simulink model "controle_pid"  (R2018b)
settings: Solver=VariableStepAuto  StartTime=0.0  StopTime=800  RelTol=1e-3
values from neighbouring files (symbols this model uses):
  h10 = 25    [dadosTanque.m]
  h20 = 20    [dadosTanque.m]
  k1 = 25    [dadosTanque.m]
  k2 = 25    [dadosTanque.m]
  kac = 20    [dadosTanque.m]
  Ki = blkdiag(Ki,1/tau(i))    [calcula_parametros_PID.m]
  Kp = blkdiag(Kp, 0.6*tau(i)/(k(i)*theta(i)))    [calcula_parametros_PID.m]
  q10 = k1*sqrt(h10) + kac*sqrt(h10-h20)    [dadosTanque.m]
  q20 = k2*sqrt(h20) - kac*sqrt(h10-h20)    [dadosTanque.m]
  sw_anti_windup = 1    [simula_anti_windup.m]    (also in simula_d_filter.m; simula_noise.m; simula_pid.m = 0)
  sw_d_filter = 0    [simula_anti_windup.m]    (also in simula_d_filter.m = 1; simula_noise.m; simula_pid.m)
  sw_noise = 0    [simula_anti_windup.m]    (also in simula_d_filter.m = 1; simula_div_acao_pond.m = 1; simula_div_acao_pond2.m = 1; simula_div_acao_trad.m = 1)
  Td = blkdiag(Td,theta(i)/2)    [calcula_parametros_PID.m]
settings Model: Creator=Caléo  LastModifiedBy=Caléo
settings SolverCC: ZeroCrossAlgorithm=Adaptive
settings DebuggingCC: IgnoredZcDiagnostic=none

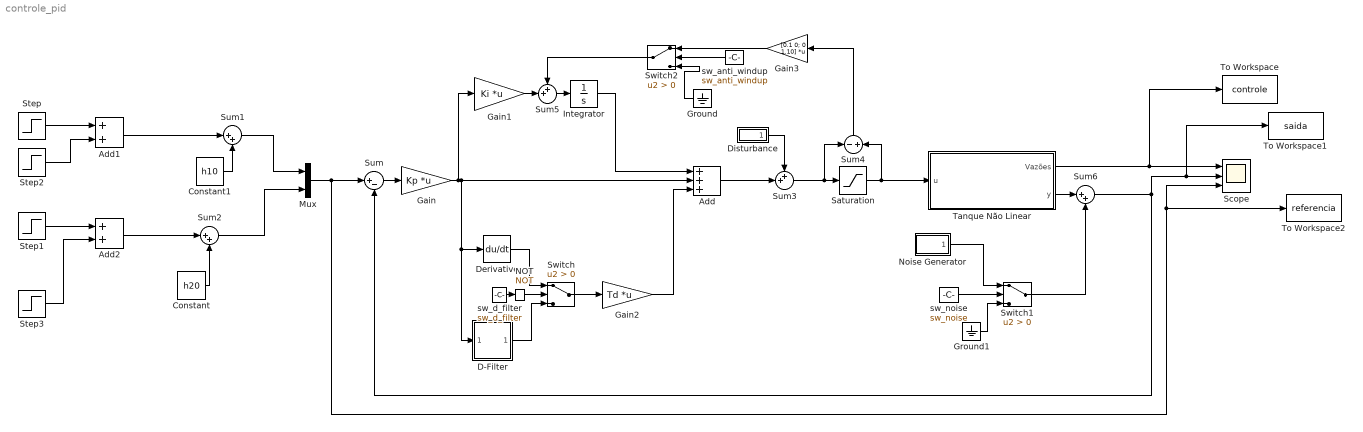
== system controle_pid ==
  Add : Sum  Inputs=+++
  Add1 : Sum
  Add2 : Sum
  Constant : Constant  Value=h20
  Constant1 : Constant  Value=h10
  D-Filter : Subsystem
  Derivative : Derivative
  Disturbance : Subsystem
  Gain : Gain  Gain=Kp  Multiplication=Matrix(K*u)
  Gain1 : Gain  Gain=Ki  Multiplication=Matrix(K*u)
  Gain2 : Gain  Gain=Td  Multiplication=Matrix(K*u)
  Gain3 : Gain  Gain=[0.1 0; 0 1.10]  Multiplication=Matrix(K*u)
  Ground : Ground
  Ground1 : Ground
  Integrator : Integrator
  Mux : Mux  Inputs=2
  NOT : Logic  Operator=NOT  IconShape=distinctive  AllPortsSameDT=off  OutDataTypeStr=boolean
  Noise Generator : Subsystem
  Saturation : Saturate  UpperLimit=[0.2*q10 0.2*q20]  LowerLimit=[-q10 ;-q20]
  Scope : Scope  NumInputPorts=3
  Step : Step  After=5  SampleTime=0
  Step1 : Step  After=3  SampleTime=0
  Step2 : Step  Time=300  After=-6  SampleTime=0
  Step3 : Step  Time=300  After=-6  SampleTime=0
  Sum : Sum  Inputs=|+-
  Sum1 : Sum  Inputs=|++
  Sum2 : Sum  Inputs=|++
  Sum3 : Sum  Inputs=++|
  Sum4 : Sum  Inputs=-+
  Sum5 : Sum  Inputs=++|
  Sum6 : Sum  Inputs=|++
  Switch : Switch  Criteria=u2 > Threshold
  Switch1 : Switch  Criteria=u2 > Threshold
  Switch2 : Switch  Criteria=u2 > Threshold
  Tanque Não Linear : Subsystem
  To Workspace : ToWorkspace  VariableName=controle  SaveFormat=Timeseries  SampleTime=-1
  To Workspace1 : ToWorkspace  VariableName=saida  SaveFormat=Timeseries  SampleTime=-1
  To Workspace2 : ToWorkspace  VariableName=referencia  SaveFormat=Timeseries  SampleTime=-1
  sw_anti_windup : Constant  Value=sw_anti_windup
  sw_d_filter : Constant  Value=sw_d_filter
  sw_noise : Constant  Value=sw_noise
  wires:
  Gain/1 -> Derivative/1, D-Filter/1(In1), Add/2, Gain1/1
  Mux/1 -> To Workspace2/1, Scope/3, Sum/1
  Sum/1 -> Gain/1
  Constant/1 -> Sum2/2
  Constant1/1 -> Sum1/2
  Sum1/1 -> Mux/1
  Sum2/1 -> Mux/2
  Tanque Não Linear/1(Vazões) -> To Workspace/1, Scope/1
  Step/1 -> Add1/1
  Step2/1 -> Add1/2
  Step1/1 -> Add2/1
  Step3/1 -> Add2/2
  Add2/1 -> Sum2/1
  Add1/1 -> Sum1/1
  Sum3/1 -> Sum4/1, Saturation/1
  Saturation/1 -> Tanque Não Linear/1(u), Sum4/2
  Integrator/1 -> Add/1
  Sum4/1 -> Gain3/1
  Gain1/1 -> Sum5/2
  Sum5/1 -> Integrator/1
  Gain3/1 -> Switch2/1
  Switch2/1 -> Sum5/1
  Ground/1 -> Switch2/3
  Tanque Não Linear/2(y) -> Sum6/1
  Ground1/1 -> Switch1/3
  Sum6/1 -> Sum/2, To Workspace1/1, Scope/2
  Gain2/1 -> Add/3
  Add/1 -> Sum3/2
  Disturbance/1(Out1) -> Sum3/1
  sw_noise/1 -> Switch1/2
  sw_anti_windup/1 -> Switch2/2
  Noise Generator/1(Out1) -> Switch1/1
  Switch/1 -> Gain2/1
  D-Filter/1(Out1) -> Switch/3
  Derivative/1 -> Switch/1
  sw_d_filter/1 -> NOT/1
  NOT/1 -> Switch/2
  Switch1/1 -> Sum6/2

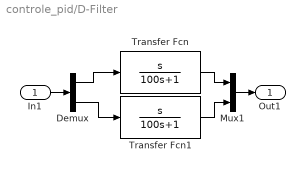
== system controle_pid/D-Filter ==
  In1 : Inport
  Demux : Demux  Outputs=2
  Mux1 : Mux  Inputs=2
  Transfer Fcn : TransferFcn  Numerator=[1 0]  Denominator=[100 1]
  Transfer Fcn1 : TransferFcn  Numerator=[1 0]  Denominator=[100 1]
  Out1 : Outport
  wires:
  In1/1 -> Demux/1
  Demux/1 -> Transfer Fcn/1
  Transfer Fcn/1 -> Mux1/1
  Transfer Fcn1/1 -> Mux1/2
  Mux1/1 -> Out1/1
  Demux/2 -> Transfer Fcn1/1

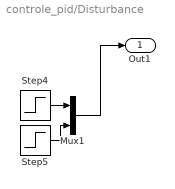
== system controle_pid/Disturbance ==
  Mux1 : Mux  Inputs=2
  Step4 : Step  Time=600  After=10  SampleTime=0
  Step5 : Step  Time=600  After=10  SampleTime=0
  Out1 : Outport
  wires:
  Step5/1 -> Mux1/2
  Mux1/1 -> Out1/1
  Step4/1 -> Mux1/1

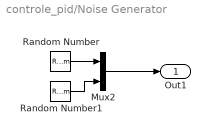
== system controle_pid/Noise Generator ==
  Mux2 : Mux  Inputs=2
  Random Number : RandomNumber  Variance=0.01  SampleTime=0.1
  Random Number1 : RandomNumber  Variance=0.01  SampleTime=0.1
  Out1 : Outport
  wires:
  Random Number1/1 -> Mux2/2
  Random Number/1 -> Mux2/1
  Mux2/1 -> Out1/1

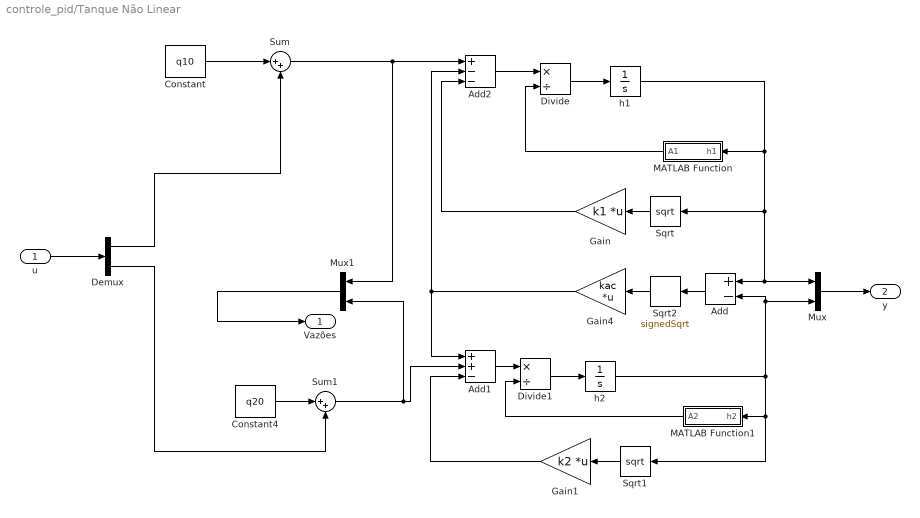
== system controle_pid/Tanque Não Linear ==
  u : Inport
  Add : Sum  Inputs=+-
  Add1 : Sum  Inputs=++-
  Add2 : Sum  Inputs=+--
  Constant : Constant  Value=q10
  Constant4 : Constant  Value=q20
  Demux : Demux  Outputs=2
  Divide : Product  Inputs=*/
  Divide1 : Product  Inputs=*/
  Gain : Gain  Gain=k1  Multiplication=Matrix(K*u)
  Gain1 : Gain  Gain=k2  Multiplication=Matrix(K*u)
  Gain4 : Gain  Gain=kac  Multiplication=Matrix(K*u)
  MATLAB Function : MATLAB Function  TreatAsAtomicUnit=on
  MATLAB Function1 : MATLAB Function  TreatAsAtomicUnit=on
  Mux : Mux  Inputs=2
  Mux1 : Mux  Inputs=2
  Sqrt : Sqrt  SaturateOnIntegerOverflow=on
  Sqrt1 : Sqrt  SaturateOnIntegerOverflow=on
  Sqrt2 : Sqrt  Operator=signedSqrt  SaturateOnIntegerOverflow=on
  Sum : Sum  Inputs=|++
  Sum1 : Sum  Inputs=|++
  h1 : Integrator  InitialCondition=h10  LimitOutput=on  UpperSaturationLimit=50  LowerSaturationLimit=0
  h2 : Integrator  InitialCondition=h20  LimitOutput=on  UpperSaturationLimit=50  LowerSaturationLimit=0
  Vazões : Outport
  y : Outport  Port=2
  wires:
  u/1 -> Demux/1
  h2/1 -> Add/2, Mux/2, MATLAB Function1/1(h2), Sqrt1/1
  Sqrt2/1 -> Gain4/1
  Gain/1 -> Add2/3
  Demux/1 -> Sum/2
  Demux/2 -> Sum1/2
  Divide/1 -> h1/1
  h1/1 -> Mux/1, Add/1, Sqrt/1, MATLAB Function/1(h1)
  Add/1 -> Sqrt2/1
  Mux1/1 -> Vazões/1
  Gain4/1 -> Add2/2, Add1/1
  Sqrt1/1 -> Gain1/1
  Constant/1 -> Sum/1
  Divide1/1 -> h2/1
  Constant4/1 -> Sum1/1
  Add1/1 -> Divide1/1
  MATLAB Function1/1(A2) -> Divide1/2
  Add2/1 -> Divide/1
  MATLAB Function/1(A1) -> Divide/2
  Gain1/1 -> Add1/3
  Mux/1 -> y/1
  Sqrt/1 -> Gain/1
  Sum/1 -> Mux1/1, Add2/1
  Sum1/1 -> Mux1/2, Add1/2

== matlab function controle_pid/Tanque Não Linear/MATLAB Function1 ==
  data: h2 input; A2 output
function A2 = secao_tanque(h2)

    if h2 < 7.5
        d2 = 6; 
    elseif h2 < 19.5
        d2 = (19.5 - h2)/2;
    elseif h2 < 29.5
        d2 = 0;
    elseif h2 < 41.5
        d2=(h2 - 29.5)/2;
    elseif h2 >= 41.5
        d2 = 6;
    else 
        d2 = 6;
    end
    A2 = 9*(14+d2);
    
end

== matlab function controle_pid/Tanque Não Linear/MATLAB Function ==
  data: h1 input; A1 output
function A1 = secao_tanque(h1)

    if h1 < 7.5
        d1 = 0;
    elseif h1 < 19.5
        d1 = (h1 - 7.5)/2;
    elseif h1 < 29.5
        d1 = 6;
    elseif h1 < 41.5
        d1 = (41.5 - h1)/2;
    elseif h1 >= 41.5
        d1 = 0;
    else 
        d1 = 0;
    end
    A1 = 9*(8+d1);
end
